simulink model "untitled"  (R2015a)
settings: Solver=ode45  StartTime=0.0  StopTime=10.0  RelTol=1e-3
values from neighbouring files (symbols this model uses):
  b = 0.55/2    (= 0.275)    [Parameters.m]
  Kq = Cq*ro*A*R^3    (= 2.88925724261e-07)    [Parameters.m]
  Kt = Ct*ro*A*R^2    (= 2.46191978476e-05)    [Parameters.m]
  x1 = [m q]    [Parameters.m]
undefined symbols (not defined in the file or in its folder): m_servo, omega_hover, q_servo
settings Model: Creator=Claudio  LastModifiedBy=Claudio

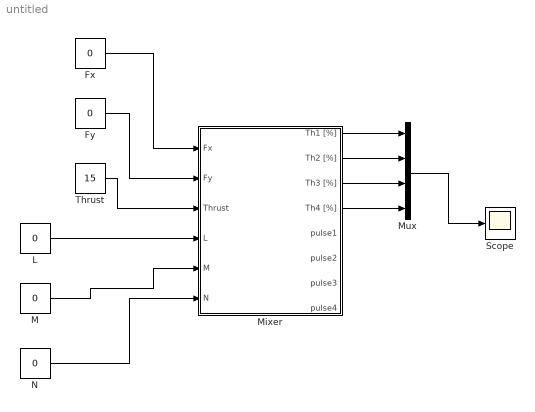
== system untitled ==
  Fx : Constant  Value=0
  Fy : Constant  Value=0
  L : Constant  Value=0
  M : Constant  Value=0
  Mixer : Subsystem  InitFcn=|
      | %%Parameters definition
      | b = 0.55/2;
      | RPMmax = 3*4.2*710;
      | D = 12*2.54/100;
      | Ct = 0.001;
      | Cq = 0.001;
      | ro = 1.225;
      | 
      | %% From omega squared to forces/torques
      |  A = ro*D^4*diag([Ct b/sqrt(2)*Ct b/sqrt(2)*Ct Cq*D]);
      |  B = [ 1  1  1 1;
      |          1 -1 -1 1;
      |         -1 -1  1 1;
      |         -1  1 -1 1];
      |  C = inv(A*B);       %TM = C * omegasq
  Mux : Mux
  N : Constant  Value=0
  Scope : Scope
  Thrust : Constant  Value=15
  wires:
  Mixer/4(Th4 [%]) -> Mux/4
  Mixer/3(Th3 [%]) -> Mux/3
  Mixer/2(Th2 [%]) -> Mux/2
  Mixer/1(Th1 [%]) -> Mux/1
  Mux/1 -> Scope/1
  Fx/1 -> Mixer/1(Fx)
  Fy/1 -> Mixer/2(Fy)
  Thrust/1 -> Mixer/3(Thrust)
  L/1 -> Mixer/4(L)
  M/1 -> Mixer/5(M)
  N/1 -> Mixer/6(N)

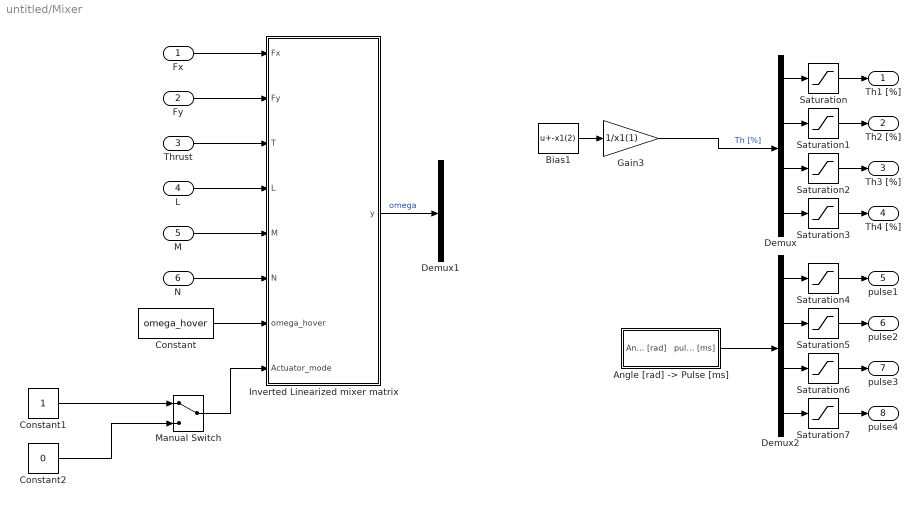
== system untitled/Mixer ==
  Fx : Inport
  Fy : Inport  Port=2
  Thrust : Inport  Port=3
  L : Inport  Port=4
  M : Inport  Port=5
  N : Inport  Port=6
  "Angle [rad] -> Pulse [ms]" : Subsystem
  Bias1 : Bias  Bias=-x1(2)
  Constant : Constant  Value=omega_hover
  Constant1 : Constant
  Constant2 : Constant  Value=0
  Demux : Demux
  Demux1 : Demux  Outputs=6
  Demux2 : Demux
  Gain3 : Gain  Gain=1/x1(1)
  Inverted Linearized mixer matrix : MATLAB Function  TreatAsAtomicUnit=on
  Manual Switch : ManualSwitch
  Saturation{,1..3} (4 alike) : Saturate  UpperLimit=100  LowerLimit=0
  Saturation{4..7} (4 alike) : Saturate  UpperLimit=2000  LowerLimit=0
  Th1 [%] : Outport
  Th2 [%] : Outport  Port=2
  Th3 [%] : Outport  Port=3
  Th4 [%] : Outport  Port=4
  pulse1 : Outport  Port=5
  pulse2 : Outport  Port=6
  pulse3 : Outport  Port=7
  pulse4 : Outport  Port=8
  wires:
  Demux/1 -> Saturation/1
  Saturation/1 -> Th1 [%]/1
  Demux/2 -> Saturation1/1
  Demux/3 -> Saturation2/1
  Demux/4 -> Saturation3/1
  Saturation3/1 -> Th4 [%]/1
  Saturation2/1 -> Th3 [%]/1
  Saturation1/1 -> Th2 [%]/1
  Gain3/1 -> Demux/1  "Th [%]"
  Bias1/1 -> Gain3/1
  Demux2/1 -> Saturation4/1
  Saturation4/1 -> pulse1/1
  Demux2/2 -> Saturation5/1
  Demux2/3 -> Saturation6/1
  Demux2/4 -> Saturation7/1
  Saturation7/1 -> pulse4/1
  Saturation6/1 -> pulse3/1
  Saturation5/1 -> pulse2/1
  Constant/1 -> Inverted Linearized mixer matrix/7(omega_hover)
  "Angle [rad] -> Pulse [ms]"/1(pulse [ms]) -> Demux2/1
  Manual Switch/1 -> Inverted Linearized mixer matrix/8(Actuator_mode)
  Constant1/1 -> Manual Switch/1
  Constant2/1 -> Manual Switch/2
  Fx/1 -> Inverted Linearized mixer matrix/1(Fx)
  Fy/1 -> Inverted Linearized mixer matrix/2(Fy)
  Thrust/1 -> Inverted Linearized mixer matrix/3(T)
  L/1 -> Inverted Linearized mixer matrix/4(L)
  M/1 -> Inverted Linearized mixer matrix/5(M)
  N/1 -> Inverted Linearized mixer matrix/6(N)
  Inverted Linearized mixer matrix/1(y) -> Demux1/1  "omega"

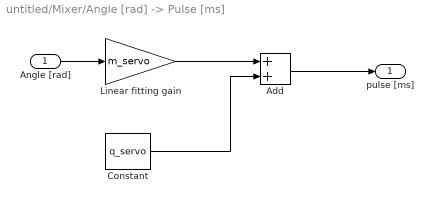
== system untitled/Mixer/Angle [rad] -> Pulse [ms] ==
  Angle [rad] : Inport
  Add : Sum
  Constant : Constant  Value=q_servo
  Linear fitting gain : Gain  Gain=m_servo
  pulse [ms] : Outport
  wires:
  Angle [rad]/1 -> Linear fitting gain/1
  Constant/1 -> Add/2
  Linear fitting gain/1 -> Add/1
  Add/1 -> pulse [ms]/1

== matlab function untitled/Mixer/Inverted Linearized mixer matrix ==
  data: Fx input; Fy input; T input; L input; M input; N input; y output; omega_hover input; Kt parameter; Kq parameter; b parameter; Actuator_mode input
function y = fcn(Fx,Fy,T,L,M,N,omega_hover,Kt,Kq,b,Actuator_mode)
%#codegen

%input column vector
u = [Fx;Fy;T;L;M;N];

omega_1sq = omega_hover^2;
omega_2sq = omega_hover^2;
omega_3sq = omega_hover^2;
omega_4sq = omega_hover^2;

% Linearided "mixer matrix" evaluated in a hover condition

% J_at_hover =[                   0,    2*Kt*omega_hover,                   0,   -2*Kt*omega_hover,                   0,                  0,                  0,                   0;
%    -2*Kt*omega_hover,                   0,    2*Kt*omega_hover,                   0,                   0,                  0,                  0,                   0;
%                    0,                   0,                   0,                   0,    Kt*omega_hover^2,   Kt*omega_hover^2,   Kt*omega_hover^2,    Kt*omega_hover^2;
%                    0,    2*Kq*omega_hover,                   0,   -2*Kq*omega_hover,                   0, Kt*b*omega_hover^2,                  0, -Kt*b*omega_hover^2;
%     2*Kq*omega_hover,                   0,   -2*Kq*omega_hover,                   0, -Kt*b*omega_hover^2,                  0, Kt*b*omega_hover^2,                   0;
%  -2*Kt*b*omega_hover, -2*Kt*b*omega_hover, -2*Kt*b*omega_hover, -2*Kt*b*omega_hover,   -Kq*omega_hover^2,   Kq*omega_hover^2,  -Kq*omega_hover^2,    Kq*omega_hover^2]
 
% switch Actuator_mode
%     case 1  % Fixed alpha - Normal quadrotor
%         Mixer_matrix = [-Kt -Kt -Kt -Kt; 0 -Kt*b 0 Kt*b;Kt*b 0 -Kt*b 0 ; Kq -Kq Kq -Kq]
%         Mix_mat_inv = Mixer_matrix^-1;
%         result_ = Mix_mat_inv*[L;M;N;T];
%         
%     case 2
%         %Jinv = pinv(J_at_hover);
%         result_= [ 0; 0 ; 0 ; 0];
% end
 
%Jinv = pinv(J_at_hover);

MM= [    0,     0,     0,    0,                               0,   - Kt*omega_2sq - Kt*omega_4sq;
    0,     0,     0,    0,     Kt*omega_1sq + Kt*omega_3sq,                               0;
  -Kt,   -Kt,   -Kt,  -Kt,                               0,                               0;
    0, -Kt*b,     0, Kt*b,                               0,   - Kq*omega_2sq - Kq*omega_4sq;
 Kt*b,     0, -Kt*b,    0,   - Kq*omega_1sq - Kq*omega_3sq,                               0;
   Kq,   -Kq,    Kq,  -Kq, Kt*b*omega_1sq - Kt*b*omega_3sq, Kt*b*omega_2sq - Kt*b*omega_4sq]



y = MM*u;
